simulink model "SmoothStepTest"  (R2016b)
settings: Solver=FixedStepAuto  StartTime=0.0  StopTime=1000  FixedStep=0.002  RelTol=1e-3
settings Model: Creator=march  LastModifiedBy=march

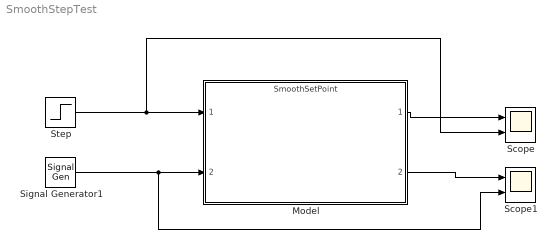
== system SmoothStepTest ==
  Model : ModelReference  ModelNameDialog=SmoothSetPoint.slx  SimulationMode=Normal  ModelReferenceVersion=1.62
  Scope : Scope  NumInputPorts=2
  Scope1 : Scope  NumInputPorts=2
  Signal Generator1 : SignalGenerator  WaveForm=square  Amplitude=5  Frequency=0.02  Units=rad/sec
  Step : Step  After=100
  wires:
  Model/1 -> Scope/1
  Step/1 -> Scope/2, Model/1
  Signal Generator1/1 -> Scope1/2, Model/2
  Model/2 -> Scope1/1
